simulink model "simulink_model"  (R2024a)
settings: Solver=VariableStepAuto  StartTime=0.0  StopTime=10.0  RelTol=1e-3
values from neighbouring files (symbols this model uses):
  A1 = [0, K/(Jt); -K/(L), -R/L]    [cp1_startup.m]
  B1 = [0; 1/L]    [cp1_startup.m]
  C1 = [1, 0]    [cp1_startup.m]
  K = Tildek*TildeWr*inv(Wr)    [cp1_startup.m]
  k_r = -1/(C1*inv(A1-B1*K)*B1)    [cp1_startup.m]
settings Model: Creator=lauramariaquirosconesa  LastModifiedBy=lauramariaquirosconesa

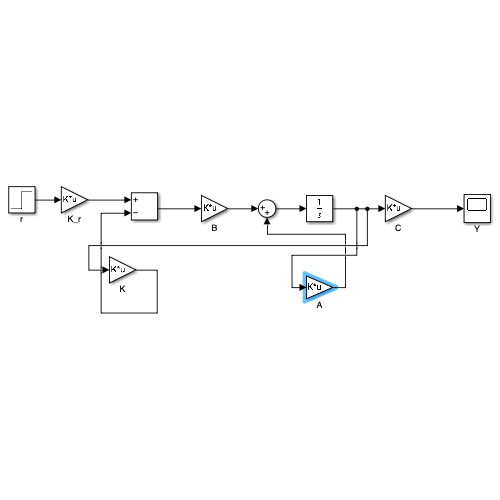
[thumbnail: Simulink's stored preview of the top-level diagram]
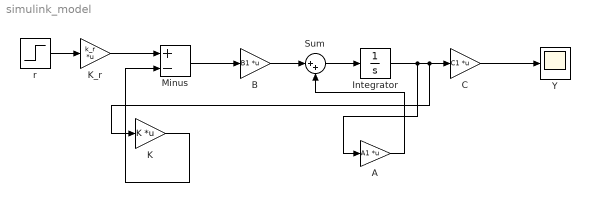
== system simulink_model ==
  A : Gain  Gain=A1  Multiplication=Matrix(K*u)
  B : Gain  Gain=B1  Multiplication=Matrix(K*u)
  C : Gain  Gain=C1  Multiplication=Matrix(K*u)
  Integrator : Integrator
  K : Gain  Gain=K  Multiplication=Matrix(K*u)
  K_r : Gain  Gain=k_r  Multiplication=Matrix(K*u)
  Minus : Sum  Inputs=+-
  Sum : Sum  Inputs=|++
  Y : Scope
  r : Step  SampleTime=0
  wires:
  Integrator/1 -> A/1, K/1, C/1
  A/1 -> Sum/2
  Sum/1 -> Integrator/1
  B/1 -> Sum/1
  C/1 -> Y/1
  Minus/1 -> B/1
  K/1 -> Minus/2
  K_r/1 -> Minus/1
  r/1 -> K_r/1
